simulink model "Peregrine_falcon_near_surface"  (R2025b)
settings: Solver=VariableStepAuto  StartTime=0.0  StopTime=2.5  RelTol=1e-3
undefined symbols (not defined in the file): A1, A2, Cd1, Cd2, g, m, rho
settings Model: Creator=User  LastModifiedBy=User

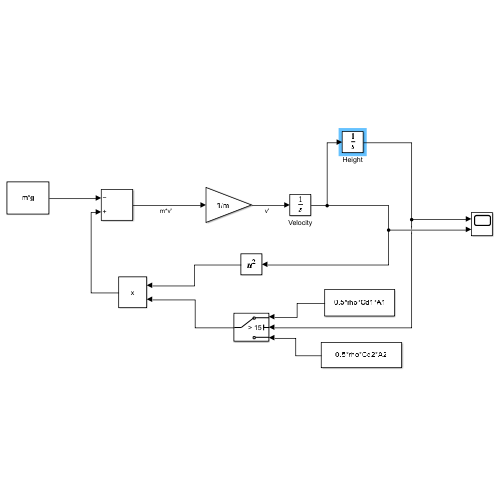
[thumbnail: Simulink's stored preview of the top-level diagram]
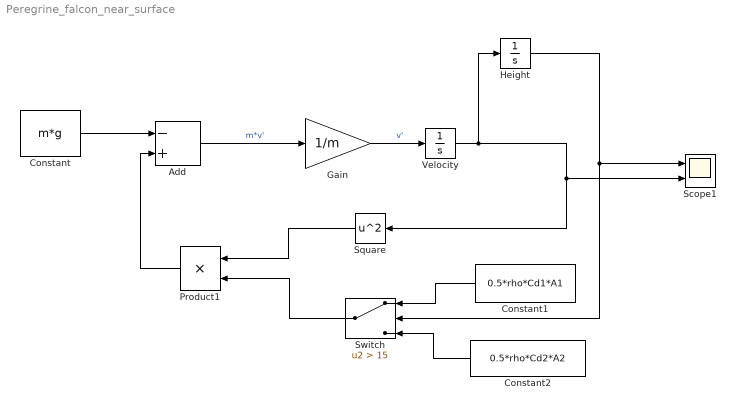
== system Peregrine_falcon_near_surface ==
  Add : Sum  Inputs=-+
  Constant : Constant  Value=m*g
  Constant1 : Constant  Value=0.5*rho*Cd1*A1
  Constant2 : Constant  Value=0.5*rho*Cd2*A2
  Gain : Gain  Gain=1/m
  Height : Integrator  InitialCondition=60
  Product1 : Product
  Scope1 : Scope  NumInputPorts=2
      settings: ActiveDisplayYMinimum=-42.207018381142525  ActiveDisplayYMaximum=71.3563353756825
  Square : Math  Operator=square
  Switch : Switch  Criteria=u2 > Threshold  Threshold=15  SaturateOnIntegerOverflow=off  InputSameDT=off
  Velocity : Integrator  InitialCondition=-10
  wires:
  Constant/1 -> Add/1
  Product1/1 -> Add/2
  Switch/1 -> Product1/2
  Square/1 -> Product1/1
  Constant1/1 -> Switch/1
  Constant2/1 -> Switch/3
  Add/1 -> Gain/1  "m*v'"
  Gain/1 -> Velocity/1  "v'"
  Velocity/1 -> Height/1, Scope1/2, Square/1
  Height/1 -> Switch/2, Scope1/1
